simulink model "port_checker_2014B"  (R2014b)
settings: Solver=ode45  StartTime=0.0  StopTime=10  RelTol=1e-3
libraries: dspnetwork x8, rtwinlib x1
settings Model: CovModelRefEnable=off  CovSFcnEnable=on  Creator=dave  LastModifiedBy=petrhomolka
settings DataIOCC: SaveFormat=StructureWithTime
settings DebuggingCC: SolverPrmCheckMsg=none  FrameProcessingCompatibilityMsg=error
settings HardwareCC: ProdBitPerPointer=64  ProdLargestAtomicFloat=Float  ProdIntDivRoundTo=Zero  ProdEndianess=LittleEndian  ProdHWDeviceType=Specified
settings GRTTargetCC: GeneratePreprocessorConditionals=Use local settings

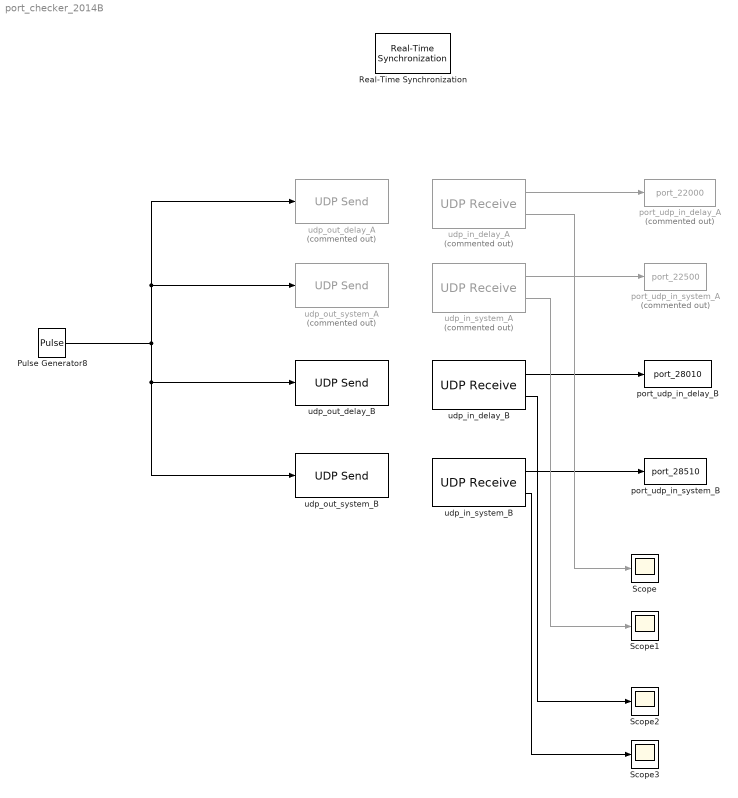
== system port_checker_2014B ==
  Pulse Generator8 : DiscretePulseGenerator  PulseType=Time based  Period=1  PulseWidth=5
  Real-Time Synchronization : rtwinlib/Real-Time Synchronization  SampleTime=0.1  MaxMissedTicks=inf  ShowMissedTicks=off  YieldWhenWaiting=off
  Scope{,1..3} (4 alike) : Scope
      Scope settings: TimeRange=auto  LimitDataPoints=on  MaxDataPoints=5000  SaveToWorkspace=off  SaveName=ScopeData  YMin=-10  YMax=10  SampleTime=-1  DataFormat=Array
      Scope1 settings: TimeRange=auto  LimitDataPoints=on  MaxDataPoints=5000  SaveToWorkspace=off  YMin=-10  YMax=10  SampleTime=-1  DataFormat=Array
      Scope2 settings: TimeRange=auto  LimitDataPoints=on  MaxDataPoints=5000  SaveToWorkspace=off  SaveName=ScopeData2  YMin=-10  YMax=10  SampleTime=-1  DataFormat=Array
      Scope3 settings: TimeRange=auto  LimitDataPoints=on  MaxDataPoints=5000  SaveToWorkspace=off  SaveName=ScopeData3  YMin=-10  YMax=10  SampleTime=-1  DataFormat=Array
  port_udp_in_delay_A : ToWorkspace  Commented=on  VariableName=port_22000  SaveFormat=Timeseries  SampleTime=-1
  port_udp_in_delay_B : ToWorkspace  VariableName=port_28010  SaveFormat=Timeseries  SampleTime=-1
  port_udp_in_system_A : ToWorkspace  Commented=on  VariableName=port_22500  SaveFormat=Timeseries  SampleTime=-1
  port_udp_in_system_B : ToWorkspace  VariableName=port_28510  SaveFormat=Timeseries  SampleTime=-1
  udp_in_delay_A : dspnetwork/UDP Receive  Commented=on  localURL='0.0.0.0'  localPort=22000  remoteURL='129.10.131.51'  remotePort=-1  recvBufferSize=8192  dims=255  signalDatatype=int8  isVarSize=off  showBlockingTime=off  blockingTime=0  sampletime=0.1
  udp_in_delay_B : dspnetwork/UDP Receive  localURL='0.0.0.0'  localPort=28010  remoteURL='129.10.131.51'  remotePort=-1  recvBufferSize=8192  dims=255  signalDatatype=int8  isVarSize=off  showBlockingTime=off  blockingTime=0  sampletime=0.1
  udp_in_system_A : dspnetwork/UDP Receive  Commented=on  localURL='0.0.0.0'  localPort=22500  remoteURL='129.10.131.51'  remotePort=-1  recvBufferSize=8192  dims=255  signalDatatype=int8  isVarSize=off  showBlockingTime=off  blockingTime=0  sampletime=0.1
  udp_in_system_B : dspnetwork/UDP Receive  localURL='0.0.0.0'  localPort=28510  remoteURL='129.10.131.51'  remotePort=-1  recvBufferSize=8192  dims=255  signalDatatype=int8  isVarSize=off  showBlockingTime=off  blockingTime=0  sampletime=0.1
  udp_out_delay_A : dspnetwork/UDP Send  Commented=on  remoteURL='129.10.131.51'  remotePort=23000  localURL='0.0.0.0'  localPortSource=Automatically determine  localPort=-1  sampletime=-1  separateLengthPort=0
  udp_out_delay_B : dspnetwork/UDP Send  remoteURL='129.10.131.51'  remotePort=27010  localURL='0.0.0.0'  localPortSource=Automatically determine  localPort=-1  sampletime=-1  separateLengthPort=0
  udp_out_system_A : dspnetwork/UDP Send  Commented=on  remoteURL='129.10.131.51'  remotePort=23500  localURL='0.0.0.0'  localPortSource=Automatically determine  localPort=-1  sampletime=-1  separateLengthPort=0
  udp_out_system_B : dspnetwork/UDP Send  remoteURL='129.10.131.51'  remotePort=27510  localURL='0.0.0.0'  localPortSource=Automatically determine  localPort=-1  sampletime=-1  separateLengthPort=0
  wires:
  Pulse Generator8/1 -> udp_out_system_B/1, udp_out_delay_B/1, udp_out_system_A/1, udp_out_delay_A/1
  udp_in_delay_A/1 -> port_udp_in_delay_A/1
  udp_in_system_B/1 -> port_udp_in_system_B/1
  udp_in_delay_B/1 -> port_udp_in_delay_B/1
  udp_in_system_A/1 -> port_udp_in_system_A/1
  udp_in_delay_A/2 -> Scope/1
  udp_in_system_A/2 -> Scope1/1
  udp_in_delay_B/2 -> Scope2/1
  udp_in_system_B/2 -> Scope3/1
